simulink model "Modelo_COMPLETO_MARTIN"  (R2021a)
settings: Solver=ode15s  StartTime=0.0  StopTime=100  FixedStep=0.001  MaxStep=0.0003  RelTol=1e-3
InitFcn:
  | errordlg(DAStudio.message('Stateflow:misc:CannotSimulateWithDemoLicense'));DAStudio.error('Stateflow:misc:InvalidStateflowLicense');
model workspace (MAT data in the model file):
  socvcb = containers.Map
  socvcb.serialization.keys = {}
  socvcb.serialization.values = {}
  socvcb.serialization.uniformity = 0
  socvcb.serialization.keyType = 'double'
  socvcb.serialization.valueType = 'any'
values from neighbouring files (symbols this model uses):
  a_l_max = 0.75    [WorkspaceData.m]
  a_t_max = 0.8    [WorkspaceData.m]
  b_ah = -(b_eqh/i_h - n_h*w_posh*J_eqh/i_h)    [WorkspaceData.m]
  b_at = -double(soluc.b_at)    [WorkspaceData.m]
  b_cx = 1e6    (= 1000000)    [WorkspaceData.m]
  b_cy = 1e7    (= 10000000)    [WorkspaceData.m]
  b_hb = 1.0E+8    (= 100000000)    [WorkspaceData.m]
  b_hd = 8    [WorkspaceData.m]
  b_hEb = 2.2E+9    (= 2200000000)    [WorkspaceData.m]
  b_hm = 18    [WorkspaceData.m]
  b_t = 90    [WorkspaceData.m]
  b_tb = 5e6    (= 5000000)    [WorkspaceData.m]
  b_td = 1.8    [WorkspaceData.m]
  b_tm = 6    [WorkspaceData.m]
  b_tw = 3.0e3    (= 3000)    [WorkspaceData.m]
  b_wu = 1500    [WorkspaceData.m]
  barco_x = 0:0.01:50    [WorkspaceData.m]
  barco_y = interp1(bx_c0,by_c0,barco_x,'previous')    [WorkspaceData.m]
  carro_y = ones(1,20)*45    [WorkspaceData.m]
  constante_frenos = 10    [WorkspaceData.m]
  f = 0.1    [WorkspaceData.m]
  F_D_n_x = ones(1,5)*50    [WorkspaceData.m]
  F_D_n_y = 43:1:47    [WorkspaceData.m]
  F_D_u_x = ones(1,5)*53    [WorkspaceData.m]
  F_D_u_y = 43:1:47    [WorkspaceData.m]
  F_I_n_x = ones(1,5)*-30    [WorkspaceData.m]
  F_I_n_y = 43:1:47    [WorkspaceData.m]
  F_I_u_x = ones(1,5)*-33    [WorkspaceData.m]
  F_I_u_y = 43:1:47    [WorkspaceData.m]
  g = 9.80665    [WorkspaceData.m]
  H_c = 2.5    [WorkspaceData.m]
  i_h = 22    [WorkspaceData.m]
  i_t = 30    [WorkspaceData.m]
  J_hdhEb = 3800    [WorkspaceData.m]
  J_hmhb = 30    [WorkspaceData.m]
  J_td = 1200    [WorkspaceData.m]
  J_tmtb = 7    [WorkspaceData.m]
  K_cy = 1.8e9    (= 1800000000)    [WorkspaceData.m]
  K_sah = -n_h*w_posh^2*J_eqh/i_h    [WorkspaceData.m]
  K_sat = double(soluc.K_sat)    [WorkspaceData.m]
  K_siah = w_posh^3*J_eqh/i_h    [WorkspaceData.m]
  K_siat = -double(soluc.K_siat)    [WorkspaceData.m]
  K_tw = 4.8e5    (= 480000)    [WorkspaceData.m]
  k_wu = 2.36E+9    (= 2360000000)    [WorkspaceData.m]
  M_cmax = 70000    [WorkspaceData.m]
  M_s = 15000    [WorkspaceData.m]
  M_t = 30000    [WorkspaceData.m]
  muelle_x = -35:0.01:0    [WorkspaceData.m]
  muelle_y = interp1(mx_c0,my_c0,muelle_x,'previous')    [WorkspaceData.m]
  pos_i_lh = 45-pos_i_yl    [WorkspaceData.m]
  pos_i_x = -13.5    [WorkspaceData.m]
  pos_i_yl = Y_c0(100*(pos_i_x+30)+1)+1    [WorkspaceData.m]
  r_hd = 0.75    [WorkspaceData.m]
  r_td = 0.5    [WorkspaceData.m]
  riel_x = -35:1:55    [WorkspaceData.m]
  riel_y = ones(1,91)*45    [WorkspaceData.m]
  T_hbMax = 5e4    (= 50000)    [WorkspaceData.m]
  T_hEbMax = 1.1e6    (= 1100000)    [WorkspaceData.m]
  T_s0 = T_s1    (= 0.02)    [WorkspaceData.m]
  T_s1 = 20e-3    (= 0.02)    [WorkspaceData.m]
  T_s2 = 5e-3    (= 0.005)    [WorkspaceData.m]
  T_tbmax = 5e3    (= 5000)    [WorkspaceData.m]
  tau_hm = 1e-3    (= 0.001)    [WorkspaceData.m]
  tau_tm = 1e-3    (= 0.001)    [WorkspaceData.m]
  xx_c0 = -30:0.01:50    [WorkspaceData.m]
  Y_t0 = 45    [WorkspaceData.m]
undefined symbols (not defined in the file or in its folder): sfprivate
libraries: simulink x9, vrlib x1
PreSaveFcn:
  | errordlg(DAStudio.message('Stateflow:misc:CannotSaveWithDemoLicense'));DAStudio.error('Stateflow:misc:InvalidStateflowLicense');
settings Model: Creator=Martin Tous

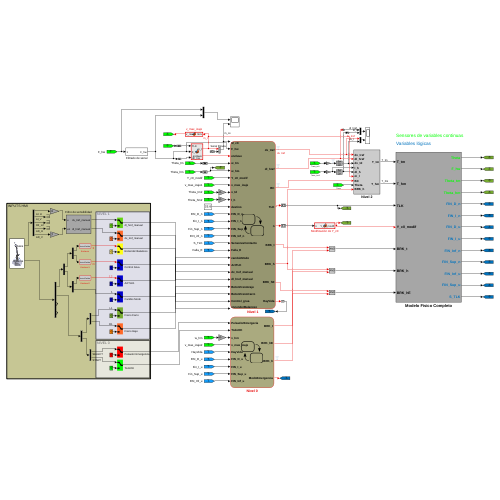
[thumbnail: Simulink's stored preview of the top-level diagram]
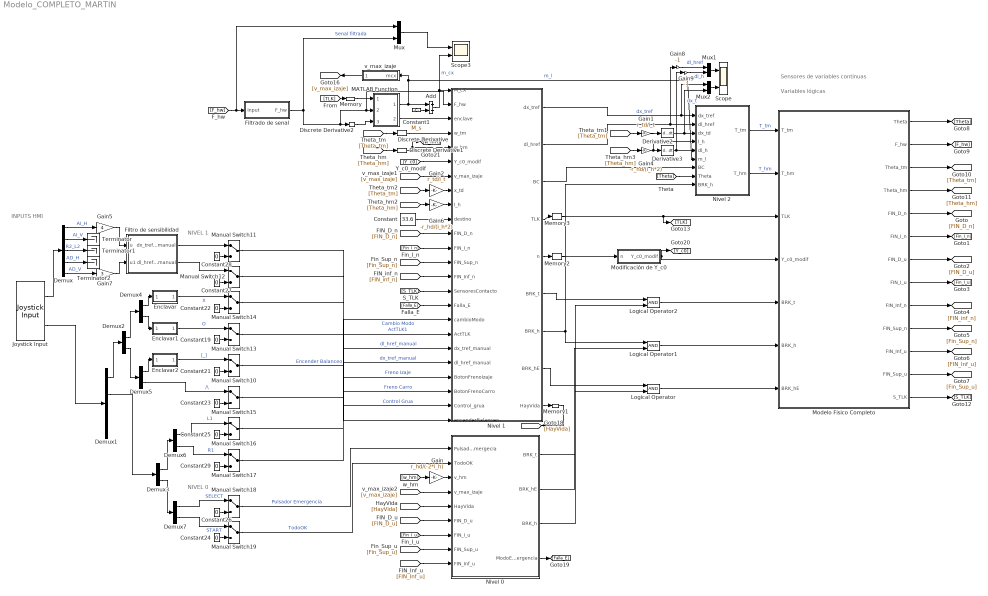
== system Modelo_COMPLETO_MARTIN ==
  note: Variables lógicas
  note: Sensores de variables continuas
  note: INPUTS HMI
  note: NIVEL 1
  note: NIVEL 0
  Add : Sum  Inputs=+-
  Constant : Constant  Value=33.6
  Constant1 : Constant  Value=M_s  SampleTime=T_s1
  Constant{19,21..23,25,27..29} (8 alike) : Constant  Value=0  SampleTime=T_s1
  Constant24 : Constant  Value=0  SampleTime=T_s0
  Constant26 : Constant  Value=0  SampleTime=T_s0
  Demux : Demux  Outputs=5
  Demux1 : Demux
  Demux{2..7} (6 alike) : Demux  Outputs=2
  Derivative2 : Derivative
  Derivative3 : Derivative
  Discrete Derivative : simulink/Discrete/Discrete Derivative  gainval=1.0  ICPrevScaledInput=0.0  OutMin=[]  OutMax=[]  OutDataType=fixdt(1, 16)  OutScaling=2^-10  DoSatur=off
  Discrete Derivative1 : simulink/Discrete/Discrete Derivative  gainval=1.0  ICPrevScaledInput=0.0  OutMin=[]  OutMax=[]  OutDataType=fixdt(1, 16)  OutScaling=2^-10  DoSatur=off
  Discrete Derivative2 : simulink/Discrete/Discrete Derivative  gainval=1.0  ICPrevScaledInput=0.0  OutMin=[]  OutMax=[]  OutDataType=fixdt(1, 16)  OutScaling=2^-10  DoSatur=off
  Enclavar : Stateflow chart  InitFcn=sfprivate('sf_demo_disclaimer');error('Preventing simulation in the absence of Stateflow license');  TreatAsAtomicUnit=on  mask(INVALID){}
      settings: PreSaveFcn=sfprivate('sf_demo_disclaimer');error('Preventing save to avoid model corruptions in the absence of Stateflow license');  OpenFcn=sfprivate('sf_demo_disclaimer');
  Enclavar1 : Stateflow chart  InitFcn=sfprivate('sf_demo_disclaimer');error('Preventing simulation in the absence of Stateflow license');  TreatAsAtomicUnit=on  mask(INVALID){}
      settings: PreSaveFcn=sfprivate('sf_demo_disclaimer');error('Preventing save to avoid model corruptions in the absence of Stateflow license');  OpenFcn=sfprivate('sf_demo_disclaimer');
  Enclavar2 : Stateflow chart  InitFcn=sfprivate('sf_demo_disclaimer');error('Preventing simulation in the absence of Stateflow license');  TreatAsAtomicUnit=on  mask(INVALID){}
      settings: PreSaveFcn=sfprivate('sf_demo_disclaimer');error('Preventing save to avoid model corruptions in the absence of Stateflow license');  OpenFcn=sfprivate('sf_demo_disclaimer');
  Filtrado de senal : Subsystem
  Filtro de sensibilidad : Subsystem
  Gain : Gain  Gain=r_hd/(-2*i_h)
  Gain1 : Gain  Gain=r_td/i_t
  Gain2 : Gain  Gain=r_td/i_t
  Gain4 : Gain  Gain=-r_hd/(i_h*2)
  Gain5 : Gain  Gain=4
  Gain6 : Gain  Gain=-r_hd/(i_h*2)
  Gain7 : Gain  Gain=3
  Gain8 : Gain  Gain=-1
  Gain9 : Gain  Gain=-1
  Joystick Input : vrlib/Joystick Input  joyid=1  adjustports=on  forcefeed=off
  Logical Operator : Logic  AllPortsSameDT=off  OutDataTypeStr=boolean
  Logical Operator1 : Logic  AllPortsSameDT=off  OutDataTypeStr=boolean
  Logical Operator2 : Logic  AllPortsSameDT=off  OutDataTypeStr=boolean
  MATLAB Function : MATLAB Function  InitFcn=sfprivate('sf_demo_disclaimer');error('Preventing simulation in the absence of Stateflow license');  TreatAsAtomicUnit=on  mask(INVALID){}
      settings: PreSaveFcn=sfprivate('sf_demo_disclaimer');error('Preventing save to avoid model corruptions in the absence of Stateflow license');  OpenFcn=sfprivate('sf_demo_disclaimer');
  Manual Switch{10..19} (10 alike) : ManualSwitch
  Memory : Memory  InheritSampleTime=on  LinearizeAsDelay=on
  Memory1 : Memory  InheritSampleTime=on
  Memory2 : Memory  InitialCondition=500  InheritSampleTime=on
  Memory3 : Memory  InheritSampleTime=on
  Modelo Fisico Completo : Subsystem
  Modificación de Y_c0 : MATLAB Function  InitFcn=sfprivate('sf_demo_disclaimer');error('Preventing simulation in the absence of Stateflow license');  TreatAsAtomicUnit=on  mask(INVALID){}
      settings: PreSaveFcn=sfprivate('sf_demo_disclaimer');error('Preventing save to avoid model corruptions in the absence of Stateflow license');  OpenFcn=sfprivate('sf_demo_disclaimer');
  Mux : Mux  Inputs=2
  Mux1 : Mux  Inputs=2
  Mux2 : Mux  Inputs=2
  Nivel 0 : Stateflow chart  InitFcn=sfprivate('sf_demo_disclaimer');error('Preventing simulation in the absence of Stateflow license');  TreatAsAtomicUnit=on  mask(INVALID){}
      settings: PreSaveFcn=sfprivate('sf_demo_disclaimer');error('Preventing save to avoid model corruptions in the absence of Stateflow license');  OpenFcn=sfprivate('sf_demo_disclaimer');  PortSchema="{\"entries\":[{\"content\":{\"sides\":[{\"content\":{\"connectorIds\":[\"In6\",\"In9\",\"In8\",\"In7\",\"In1\",\"In2\",\"In3\",\"In5\",\"In4\"]},\"type\":\"ConnectorPlacement.EquallySpacedRectSide\",\"uuid\":\"92abb5b4-7f8d-4d16-9e1c-3f1528aec02e\"},{\"content\":{\"connectorIds\":[\"Out2\",\"Out3\",\"Out1\",\"Out4\"],\"side\":\"RIGHT\"},\"type\":\"ConnectorPlacement.EquallySpacedRectSide\",\"uuid\":\"fdfc4918-925b-4492-9924-9f3ed7c6f0ea\"},{\"content\":{\"connectorIds\":[],\"side\":\"TOP\"},\"type\":\"ConnectorPlacement.EquallySpacedRectSide\",\"uuid\":\"6cd2c614-9727-439b-b51b-96ebe361e1e6\"},{\"content\":{\"connectorIds\":[],\"side\":\"BOTTOM\"},\"type\":\"ConnectorPlacement.EquallySpacedRectSide\",\"uuid\":\"c327f02f-ffd6-4494-8eea-bb6a75c04a8c\"}]},\"type\":\"ConnectorPlacement.EquallySpacedConnector\",\"uuid\":\"17c891de-27fd-4863-a62e-79c0c94ffbc9\"}],\"packageUris\":[\"http://schema.mathworks.com/mf0/Connector/R2020b\"],\"version\":\"1.0\"}"
  Nivel 1 : Stateflow chart  InitFcn=sfprivate('sf_demo_disclaimer');error('Preventing simulation in the absence of Stateflow license');  TreatAsAtomicUnit=on  mask(INVALID){}
      settings: PreSaveFcn=sfprivate('sf_demo_disclaimer');error('Preventing save to avoid model corruptions in the absence of Stateflow license');  OpenFcn=sfprivate('sf_demo_disclaimer');  PortSchema="{\"entries\":[{\"content\":{\"sides\":[{\"content\":{\"connectorIds\":[\"In1\",\"In2\",\"In23\",\"In5\",\"In4\",\"In20\",\"In13\",\"In22\",\"In21\",\"In24\",\"In7\",\"In8\",\"In10\",\"In11\",\"In3\",\"In6\",\"In19\",\"In18\",\"In9\",\"In12\",\"In15\",\"In14\",\"In16\",\"In17\"]},\"type\":\"ConnectorPlacement.EquallySpacedRectSide\",\"uuid\":\"92abb5b4-7f8d-4d16-9e1c-3f1528aec02e\"},{\"content\":{\"connectorIds\":[\"Out6\",\"Out7\",\"Out1\",\"Out8\",\"Out9\",\"Out5\",\"Out3\",\"Out4\",\"Out2\"],\"side\":\"RIGHT\"},\"type\":\"ConnectorPlacement.EquallySpacedRectSide\",\"uuid\":\"fdfc4918-925b-4492-9924-9f3ed7c6f0ea\"},{\"content\":{\"side\":\"TOP\"},\"type\":\"ConnectorPlacement.EquallySpacedRectSide\",\"uuid\":\"6cd2c614-9727-439b-b51b-96ebe361e1e6\"}]},\"type\":\"ConnectorPlacement.EquallySpacedConnector\",\"uuid\":\"17c891de-27fd-4863-a62e-79c0c94ffbc9\"}],\"packageUris\":[\"http://schema.mathworks.com/mf0/Connector/R2020b\"],\"version\":\"1.0\"}"
  Nivel 2 : Subsystem
  Scope : Scope  NumInputPorts=2
  Scope3 : Scope  NumInputPorts=2
  Terminator : Terminator
  Terminator1 : Terminator
  Terminator2 : Terminator
  v_max_izaje : MATLAB Function  InitFcn=sfprivate('sf_demo_disclaimer');error('Preventing simulation in the absence of Stateflow license');  TreatAsAtomicUnit=on  mask(INVALID){}
      settings: PreSaveFcn=sfprivate('sf_demo_disclaimer');error('Preventing save to avoid model corruptions in the absence of Stateflow license');  OpenFcn=sfprivate('sf_demo_disclaimer');
  wires:
  MATLAB Function/2(enclave) -> Nivel 1/23(enclave)
  Gain9/1 -> Mux1/2  "dl_h"
  Memory/1 -> MATLAB Function/1(TLK)
  [FIN_inf_n] -> Nivel 1/11(FIN_Inf_n)
  Mux/1 -> Scope3/1
  [Fin_Sup_n] -> Nivel 1/10(FIN_Sup_n)
  [Fin_Sup_u] -> Nivel 0/5(FIN_Sup_u)
  [FIN_Inf_u] -> Nivel 0/4(FIN_Inf_u)
  [Theta_hm] -> Gain4/1
  Modelo Fisico Completo/12(FIN_Sup_u) -> [Fin_Sup_u]
  Nivel 2/2(T_hm) -> Modelo Fisico Completo/2(T_hm)  "T_hm"
  Nivel 1/8(TLK) -> Memory3/1
  v_max_izaje/1(v_maxh) -> [v_max_izaje]
  [FIN_D_n] -> Nivel 1/7(FIN_D_n)
  [Theta_tm] -> Discrete Derivative/1
  Modelo Fisico Completo/6(FIN_I_n) -> [Fin_I_n]
  Filtrado de senal/1(F_hw) -> Nivel 1/2(F_hw), MATLAB Function/2(F_hw), Discrete Derivative2/1, Mux/2  "Senal filtrada"
  Add/1 -> Nivel 1/1(M_cX), Scope3/2  "m_cx"
  [Theta] -> Nivel 2/8(Theta)
  MATLAB Function/1(m_l) -> v_max_izaje/1(mcx), Nivel 2/6(m_l), Add/1  "m_l"
  Nivel 2/1(T_tm) -> Modelo Fisico Completo/1(T_tm)  "T_tm"
  Constant1/1 -> Add/2
  Gain6/1 -> Nivel 1/21(l_h)
  Logical Operator2/1 -> Modelo Fisico Completo/5(BRK_t)
  Discrete Derivative1/1 -> [w_hm], Nivel 1/4(w_hm)
  Nivel 1/3(BRK_h) -> Nivel 2/9(BRK_h), Logical Operator1/1
  [FIN_D_u] -> Nivel 0/2(FIN_D_u)
  Gain8/1 -> Mux1/1  "dl_href"
  Memory1/1 -> [HayVida]
  Modelo Fisico Completo/1(Theta) -> [Theta]
  [Fin_I_u] -> Nivel 0/3(FIN_I_u)
  Nivel 1/2(HayVida) -> Memory1/1
  Modelo Fisico Completo/9(FIN_Inf_n) -> [FIN_inf_n]
  Mux1/1 -> Scope/1
  Nivel 1/4(BRK_hE) -> Logical Operator/1
  Nivel 1/9(n) -> Memory2/1
  Memory2/1 -> Modificación de Y_c0/1(n)
  Gain/1 -> Nivel 0/8(v_hm)
  Nivel 0/4(ModoEmergencia) -> [Falla_E]
  Modelo Fisico Completo/8(FIN_I_u) -> [Fin_I_u]
  [Falla_E] -> Nivel 1/6(Falla_E)
  Modelo Fisico Completo/5(FIN_D_n) -> [FIN_D_n]
  [Theta_hm] -> Gain6/1
  Modelo Fisico Completo/7(FIN_D_u) -> [FIN_D_u]
  [w_hm] -> Gain/1
  [F_hw] -> Mux/1, Filtrado de senal/1(Input)
  [Fin_I_n] -> Nivel 1/8(FIN_I_n)
  Mux2/1 -> Scope/2
  [HayVida] -> Nivel 0/1(HayVida)
  Discrete Derivative2/1 -> MATLAB Function/3(dF_hw)
  [Theta_hm] -> Discrete Derivative1/1
  Modelo Fisico Completo/10(FIN_Sup_n) -> [Fin_Sup_n]
  Nivel 1/7(dl_href) -> Gain8/1, Nivel 2/2(dl_href)
  Logical Operator1/1 -> Modelo Fisico Completo/6(BRK_h)
  Nivel 0/2(BRK_t) -> Logical Operator2/2
  Memory3/1 -> [TLK], Modelo Fisico Completo/3(TLK)
  Nivel 0/1(BRK_h) -> Logical Operator/2
  [Theta_tm] -> Gain2/1
  Modelo Fisico Completo/2(F_hw) -> [F_hw]
  [Y_c0] -> Nivel 1/20(Y_c0_modif)
  Logical Operator/1 -> Modelo Fisico Completo/7(BRK_hE)
  [TLK] -> Memory/1
  Modelo Fisico Completo/4(Theta_hm) -> [Theta_hm]
  Gain1/1 -> Derivative2/1
  Nivel 1/5(BRK_t) -> Logical Operator2/1
  [S_TLK] -> Nivel 1/3(SensoresContacto)
  Modelo Fisico Completo/13(S_TLK) -> [S_TLK]
  Modelo Fisico Completo/3(Theta_tm) -> [Theta_tm]
  Modificación de Y_c0/1(Y_c0_modif) -> Modelo Fisico Completo/4(Y_c0_modif), [Y_c0]
  Discrete Derivative/1 -> Nivel 1/5(w_tm)
  Gain4/1 -> Nivel 2/4(l_h), Derivative3/1
  [v_max_izaje] -> Nivel 0/7(v_max_izaje)
  Nivel 0/3(BRK_hE) -> Logical Operator1/2
  Modelo Fisico Completo/11(FIN_Inf_u) -> [FIN_Inf_u]
  Gain2/1 -> Nivel 1/22(x_td)
  [v_max_izaje] -> Nivel 1/13(v_max_izaje)
  Nivel 1/1(BC) -> Nivel 2/7(BC)
  [Theta_tm] -> Gain1/1
  Derivative3/1 -> Gain9/1, Nivel 2/5(dl_h)
  Derivative2/1 -> Mux2/2, Nivel 2/3(dx_td)  "dx_t"
  Nivel 1/6(dx_tref) -> Mux2/1, Nivel 2/1(dx_tref)  "dx_tref"
  Manual Switch17/1 -> Nivel 1/15(BotonFrenoIzaje)  "Freno Izaje"
  Demux1/1 -> Demux2/1
  Demux2/1 -> Demux4/1
  Demux5/1 -> Enclavar2/1(boton)
  Demux/2 -> Terminator/1  "AI_V"
  Gain5/1 -> Filtro de sensibilidad/1(u)
  Demux1/2 -> Demux3/1
  Demux3/2 -> Demux7/1
  Enclavar2/1(salida) -> Manual Switch10/1  "[_]"
  Joystick Input/1 -> Demux/1
  Filtro de sensibilidad/1(dx_tref_manual) -> Manual Switch11/1
  Demux/1 -> Gain5/1  "AI_H"
  Demux4/1 -> Enclavar/1(boton)
  Manual Switch19/1 -> Nivel 0/9(TodoOK)  "TodoOK"
  Manual Switch18/1 -> Nivel 0/6(PulsadorEmergecia)  "Pulsador Emergencia"
  Constant26/1 -> Manual Switch18/2
  Demux/5 -> Gain7/1  "AD_V"
  Manual Switch14/1 -> Nivel 1/17(encenderBalanceo)  "Encender Balanceo"
  Filtro de sensibilidad/2(dl_href_manual) -> Manual Switch12/1
  Demux5/2 -> Manual Switch15/1  "/\\"
  Demux/4 -> Terminator2/1  "AD_H"
  Constant28/1 -> Manual Switch11/2
  Constant24/1 -> Manual Switch19/2
  Enclavar/1(salida) -> Manual Switch14/1  "X"
  Enclavar1/1(salida) -> Manual Switch13/1  "O"
  Demux7/2 -> Manual Switch19/1  "START"
  Demux2/2 -> Demux5/1
  Constant25/1 -> Manual Switch16/2
  Constant22/1 -> Manual Switch14/2
  Demux7/1 -> Manual Switch18/1  "SELECT"
  Constant23/1 -> Manual Switch15/2
  Constant29/1 -> Manual Switch17/2
  Demux6/2 -> Manual Switch17/1  "R1"
  Demux3/1 -> Demux6/1
  Constant27/1 -> Manual Switch12/2
  Manual Switch15/1 -> Nivel 1/19(cambioModo)  "Cambio Modo"
  Demux/3 -> Terminator1/1  "R2_L2"
  Demux6/1 -> Manual Switch16/1  "L1"
  Joystick Input/2 -> Demux1/1
  Constant19/1 -> Manual Switch13/2
  Manual Switch10/1 -> Nivel 1/18(ActTLK)  "ActTLK1"
  Manual Switch16/1 -> Nivel 1/14(BotonFrenoCarro)  "Freno Carro"
  Gain7/1 -> Filtro de sensibilidad/2(u1)
  Constant21/1 -> Manual Switch10/2
  Demux4/2 -> Enclavar1/1(boton)
  Manual Switch11/1 -> Nivel 1/9(dx_tref_manual)  "dl_href_manual"
  Manual Switch12/1 -> Nivel 1/12(dl_href_manual)  "dx_tref_manual"
  Manual Switch13/1 -> Nivel 1/16(Control_grua)  "Control Grua"
  Constant/1 -> Nivel 1/24(destino)

== system Modelo_COMPLETO_MARTIN/Filtrado de senal ==
  Input : Inport
  Leaky Integrator : Subsystem
  Moving average : Subsystem
  F_hw : Outport
  wires:
  Leaky Integrator/1(Salida) -> Moving average/1(Salida)  "pasa bajo"
  Input/1 -> Leaky Integrator/1(Entrada)  "sin filtrar"
  Moving average/1(F_hw) -> F_hw/1  "filtrada"

== system Modelo_COMPLETO_MARTIN/Filtro de sensibilidad ==
  u : Inport
  u1 : Inport  Port=2
  Compare To Constant : simulink/Logic and Bit Operations/Compare To Constant  relop=>=  const=f  OutDataTypeStr=boolean
  Compare To Constant1 : simulink/Logic and Bit Operations/Compare To Constant  relop=<=  const=-f  OutDataTypeStr=boolean
  Compare To Constant2 : simulink/Logic and Bit Operations/Compare To Constant  relop=>=  const=f  OutDataTypeStr=boolean
  Compare To Constant3 : simulink/Logic and Bit Operations/Compare To Constant  relop=<=  const=-f  OutDataTypeStr=boolean
  OR : Logic  Operator=OR  IconShape=distinctive  AllPortsSameDT=off  OutDataTypeStr=boolean
  OR1 : Logic  Operator=OR  IconShape=distinctive  AllPortsSameDT=off  OutDataTypeStr=boolean
  Product : Product
  Product1 : Product
  dx_tref_manual : Outport
  dl_href_manual : Outport  Port=2
  wires:
  u/1 -> Compare To Constant/1, Compare To Constant1/1, Product/2
  u1/1 -> Compare To Constant2/1, Compare To Constant3/1, Product1/2
  Compare To Constant1/1 -> OR/2
  Compare To Constant2/1 -> OR1/1
  Compare To Constant3/1 -> OR1/2
  OR1/1 -> Product1/1
  Compare To Constant/1 -> OR/1
  OR/1 -> Product/1
  Product/1 -> dx_tref_manual/1  "dx_tref_manual"
  Product1/1 -> dl_href_manual/1  "dl_href_manual"

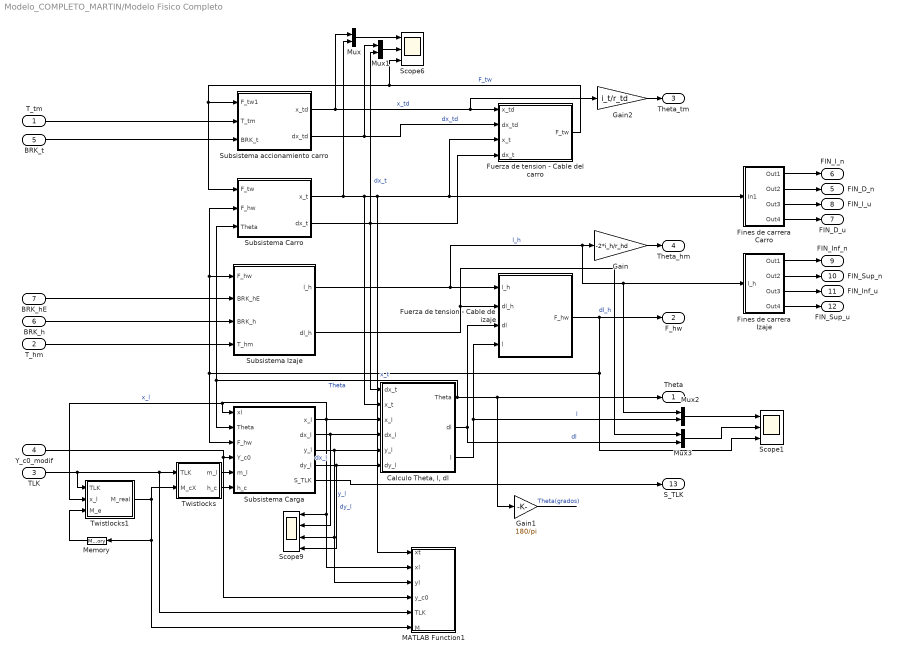
== system Modelo_COMPLETO_MARTIN/Modelo Fisico Completo ==
  T_tm : Inport
  T_hm : Inport  Port=2
  TLK : Inport  Port=3
  Y_c0_modif : Inport  Port=4
  BRK_t : Inport  Port=5
  BRK_h : Inport  Port=6
  BRK_hE : Inport  Port=7
  "Calculo Theta, l, dl" : Subsystem
  Fines de carrera Carro : Subsystem
  Fines de carrera Izaje : Subsystem
  Fuerza de tension - Cable de izaje : Subsystem
  Fuerza de tension - Cable del carro : Subsystem
  Gain : Gain  Gain=-2*i_h/r_hd
  Gain1 : Gain  Gain=180/pi
  Gain2 : Gain  Gain=i_t/r_td
  MATLAB Function1 : MATLAB Function  InitFcn=sfprivate('sf_demo_disclaimer');error('Preventing simulation in the absence of Stateflow license');  TreatAsAtomicUnit=on  mask(INVALID){}
      settings: PreSaveFcn=sfprivate('sf_demo_disclaimer');error('Preventing save to avoid model corruptions in the absence of Stateflow license');  OpenFcn=sfprivate('sf_demo_disclaimer');
  Memory : Memory  InheritSampleTime=on  LinearizeAsDelay=on
  Mux{,1..3} (4 alike) : Mux  Inputs=2
  Scope1 : Scope  NumInputPorts=3
  Scope6 : Scope  NumInputPorts=3
  Scope9 : Scope  NumInputPorts=4
  Subsistema Carga : Subsystem
  Subsistema Carro : Subsystem
  Subsistema Izaje : Subsystem
  Subsistema accionamiento carro : Subsystem
  Twistlocks : Stateflow chart  InitFcn=sfprivate('sf_demo_disclaimer');error('Preventing simulation in the absence of Stateflow license');  TreatAsAtomicUnit=on  mask(INVALID){}
      settings: PreSaveFcn=sfprivate('sf_demo_disclaimer');error('Preventing save to avoid model corruptions in the absence of Stateflow license');  OpenFcn=sfprivate('sf_demo_disclaimer');
  Twistlocks1 : Stateflow chart  InitFcn=sfprivate('sf_demo_disclaimer');error('Preventing simulation in the absence of Stateflow license');  TreatAsAtomicUnit=on  mask(INVALID){}
      settings: PreSaveFcn=sfprivate('sf_demo_disclaimer');error('Preventing save to avoid model corruptions in the absence of Stateflow license');  OpenFcn=sfprivate('sf_demo_disclaimer');  PortSchema="{\"entries\":[{\"content\":{\"sides\":[{\"content\":{\"connectorIds\":[\"In3\",\"In1\",\"In2\"]},\"type\":\"ConnectorPlacement.EquallySpacedRectSide\",\"uuid\":\"4fec8e6a-f8fa-4feb-a633-b12cd10cfa10\"},{\"content\":{\"connectorIds\":[\"Out1\"],\"side\":\"RIGHT\"},\"type\":\"ConnectorPlacement.EquallySpacedRectSide\",\"uuid\":\"3a43ccb0-d7f9-40a2-9c07-07991ad7e582\"},{\"content\":{\"connectorIds\":[],\"side\":\"TOP\"},\"type\":\"ConnectorPlacement.EquallySpacedRectSide\",\"uuid\":\"c629bb8f-87a5-4586-8b89-8bb15a2e67dc\"}]},\"type\":\"ConnectorPlacement.EquallySpacedConnector\",\"uuid\":\"e5885a79-67b0-4776-b045-dd8fc0c81e57\"}],\"packageUris\":[\"http://schema.mathworks.com/mf0/Connector/R2020b\"],\"version\":\"1.0\"}"
  Theta : Outport
  F_hw : Outport  Port=2
  Theta_tm : Outport  Port=3
  Theta_hm : Outport  Port=4
  FIN_D_n : Outport  Port=5
  FIN_I_n : Outport  Port=6
  FIN_D_u : Outport  Port=7
  FIN_I_u : Outport  Port=8
  FIN_Inf_n : Outport  Port=9
  FIN_Sup_n : Outport  Port=10
  FIN_Inf_u : Outport  Port=11
  FIN_Sup_u : Outport  Port=12
  S_TLK : Outport  Port=13
  wires:
  Fuerza de tension - Cable de izaje/1(F_hw) -> Subsistema Izaje/1(F_hw), Subsistema Carro/2(F_hw), Subsistema Carga/3(F_hw), Scope1/3, F_hw/1
  "Calculo Theta, l, dl"/1(Theta) -> Subsistema Carro/3(Theta), Subsistema Carga/2(Theta), Gain1/1, Theta/1  "Theta"
  Subsistema Izaje/2(dl_h) -> Fuerza de tension - Cable de izaje/2(dl_h), Mux3/1  "dl_h"
  Twistlocks/1(m_l) -> Subsistema Carga/5(m_l)
  "Calculo Theta, l, dl"/2(dl) -> Mux3/2, Fuerza de tension - Cable de izaje/3(dl)  "dl"
  TLK/1 -> Twistlocks/1(TLK), MATLAB Function1/5(TLK), Twistlocks1/3(TLK)
  BRK_hE/1 -> Subsistema Izaje/2(BRK_hE)
  T_hm/1 -> Subsistema Izaje/4(T_hm)
  BRK_t/1 -> Subsistema accionamiento carro/3(BRK_t)
  BRK_h/1 -> Subsistema Izaje/3(BRK_h)
  Twistlocks/2(h_c) -> Subsistema Carga/6(h_c)
  T_tm/1 -> Subsistema accionamiento carro/2(T_tm)
  Gain2/1 -> Theta_tm/1
  Subsistema Izaje/1(l_h) -> Fuerza de tension - Cable de izaje/1(l_h), Mux2/1, Fines de carrera Izaje/1(l_h), Gain/1  "l_h"
  Gain/1 -> Theta_hm/1
  "Calculo Theta, l, dl"/3(l) -> Mux2/2, Fuerza de tension - Cable de izaje/4(l)  "l"
  Twistlocks1/1(M_real) -> Memory/1, MATLAB Function1/6(M), Twistlocks/2(M_cX)
  Subsistema Carro/2(dx_t) -> Mux1/2, Fuerza de tension - Cable del carro/4(dx_t), "Calculo Theta, l, dl"/1(dx_t)  "dx_t"
  Subsistema Carga/5(S_TLK) -> S_TLK/1
  Y_c0_modif/1 -> MATLAB Function1/4(y_c0), Subsistema Carga/4(Y_c0)
  Subsistema Carro/1(x_t) -> MATLAB Function1/1(xt), Fines de carrera Carro/1(In1), Fuerza de tension - Cable del carro/3(x_t), "Calculo Theta, l, dl"/2(x_t), Mux/2  "x_t"
  Fines de carrera Carro/1(Out1) -> FIN_I_n/1
  Fines de carrera Carro/2(Out2) -> FIN_D_n/1
  Fines de carrera Carro/3(Out3) -> FIN_I_u/1
  Fines de carrera Carro/4(Out4) -> FIN_D_u/1
  Fines de carrera Izaje/1(Out1) -> FIN_Inf_n/1
  Fines de carrera Izaje/2(Out2) -> FIN_Sup_n/1
  Fines de carrera Izaje/3(Out3) -> FIN_Inf_u/1
  Fines de carrera Izaje/4(Out4) -> FIN_Sup_u/1
  Fuerza de tension - Cable del carro/1(F_tw) -> Subsistema Carro/1(F_tw), Subsistema accionamiento carro/1(F_tw1), Scope6/3  "F_tw"
  Subsistema accionamiento carro/2(dx_td) -> Mux1/1, Fuerza de tension - Cable del carro/2(dx_td)  "dx_td"
  Subsistema accionamiento carro/1(x_td) -> Gain2/1, Fuerza de tension - Cable del carro/1(x_td), Mux/1  "x_td"
  Subsistema Carga/3(y_l) -> "Calculo Theta, l, dl"/5(y_l), Scope9/3, MATLAB Function1/3(yl)  "y_l"
  Subsistema Carga/2(dx_l) -> "Calculo Theta, l, dl"/4(dx_l), Scope9/2  "dx_l"
  Subsistema Carga/4(dy_l) -> "Calculo Theta, l, dl"/6(dy_l), Scope9/4  "dy_l"
  Subsistema Carga/1(x_l) -> "Calculo Theta, l, dl"/3(x_l), Scope9/1, MATLAB Function1/2(xl), Twistlocks1/1(x_l), Subsistema Carga/1(xl)  "x_l"
  Mux/1 -> Scope6/1
  Mux1/1 -> Scope6/2
  Mux2/1 -> Scope1/1
  Mux3/1 -> Scope1/2
  Memory/1 -> Twistlocks1/2(M_e)
  Gain1/1 -> ?  "Theta(grados)"

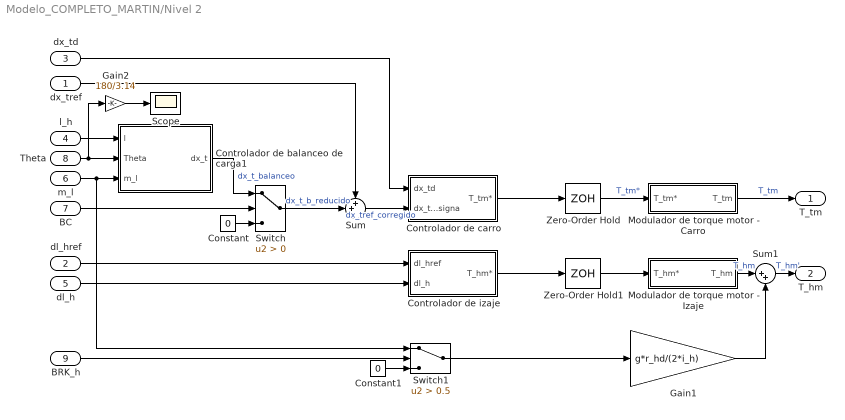
== system Modelo_COMPLETO_MARTIN/Nivel 2 ==
  dx_tref : Inport
  dl_href : Inport  Port=2
  dx_td : Inport  Port=3  SampleTime=T_s2
  l_h : Inport  Port=4  SampleTime=T_s2
  dl_h : Inport  Port=5  SampleTime=T_s2
  m_l : Inport  Port=6
  BC : Inport  Port=7
  Theta : Inport  Port=8  SampleTime=T_s2
  BRK_h : Inport  Port=9  SampleTime=T_s2
  Constant : Constant  Value=0  SampleTime=T_s2
  Constant1 : Constant  Value=0  SampleTime=T_s2
  Controlador de balanceo de carga1 : Subsystem
  Controlador de carro : Subsystem
  Controlador de izaje : Subsystem
  Gain1 : Gain  Gain=g*r_hd/(2*i_h)
  Gain2 : Gain  Gain=180/3.14
  Modulador de torque motor - Carro : Subsystem
  Modulador de torque motor - Izaje : Subsystem
  Scope : Scope
  Sum : Sum  Inputs=++|
  Sum1 : Sum  Inputs=|++
  Switch : Switch  Criteria=u2 > Threshold
  Switch1 : Switch  Criteria=u2 > Threshold  Threshold=0.5
  Zero-Order Hold : ZeroOrderHold  SampleTime=T_s2
  Zero-Order Hold1 : ZeroOrderHold  SampleTime=T_s2
  T_tm : Outport
  T_hm : Outport  Port=2
  wires:
  Sum1/1 -> T_hm/1  "T_hm'"
  Zero-Order Hold/1 -> Modulador de torque motor - Carro/1(T_tm*)  "T_tm*"
  Zero-Order Hold1/1 -> Modulador de torque motor - Izaje/1(T_hm*)
  Modulador de torque motor - Carro/1(T_tm) -> T_tm/1  "T_tm"
  Modulador de torque motor - Izaje/1(T_hm) -> Sum1/1  "T_hm"
  dx_td/1 -> Controlador de carro/1(dx_td)
  Gain2/1 -> Scope/1
  Controlador de balanceo de carga1/1(dx_t) -> Switch/1  "dx_t_balanceo"
  Theta/1 -> Controlador de balanceo de carga1/2(Theta), Gain2/1
  dx_tref/1 -> Sum/1
  Constant/1 -> Switch/3
  dl_h/1 -> Controlador de izaje/2(dl_h)
  Sum/1 -> Controlador de carro/2(dx_t_consigna)  "dx_tref_corregido"
  BC/1 -> Switch/2
  l_h/1 -> Controlador de balanceo de carga1/1(l)
  Switch/1 -> Sum/2  "dx_t_b_reducido"
  Controlador de carro/1(T_tm*) -> Zero-Order Hold/1
  Controlador de izaje/1(T_hm*) -> Zero-Order Hold1/1
  Switch1/1 -> Gain1/1
  m_l/1 -> Controlador de balanceo de carga1/3(m_l), Switch1/1
  dl_href/1 -> Controlador de izaje/1(dl_href)
  Gain1/1 -> Sum1/2
  Constant1/1 -> Switch1/3
  BRK_h/1 -> Switch1/2

== system Modelo_COMPLETO_MARTIN/Filtrado de senal/Leaky Integrator ==
  Entrada : Inport
  Constant17 : Constant
  Constant21 : Constant
  Delay1 : Delay  DelayLength=1  InitialCondition=0
  Divide1 : Product  Inputs=*/
  M : Constant  Value=100
  Product2 : Product
  Product3 : Product
  Sum3 : Sum  Inputs=-+
  Sum4 : Sum  Inputs=+-
  Sum5 : Sum  Inputs=|++
  Salida : Outport
  wires:
  Sum5/1 -> Salida/1, Delay1/1
  M/1 -> Divide1/2, Sum3/2
  Constant21/1 -> Sum4/1
  Sum4/1 -> Product2/2
  Product2/1 -> Sum5/1
  Delay1/1 -> Product3/1
  Constant17/1 -> Sum3/1
  Divide1/1 -> Product3/2, Sum4/2  "lambda"
  Product3/1 -> Sum5/2
  Sum3/1 -> Divide1/1
  Entrada/1 -> Product2/1

== system Modelo_COMPLETO_MARTIN/Filtrado de senal/Moving average ==
  Salida : Inport
  Divide : Product  Inputs=*/
  Sum of Elements : Sum  Inputs=+
  Tapped Delay : simulink/Discrete/Tapped Delay  vinit=0.0  samptime=T_s1  NumDelays=90  DelayOrder=Oldest  includeCurrent=off
  Vector Concatenate : Concatenate
  Width : Width
  F_hw : Outport
  wires:
  Width/1 -> Divide/2
  Tapped Delay/1 -> Vector Concatenate/2
  Vector Concatenate/1 -> Width/1, Sum of Elements/1
  Salida/1 -> Tapped Delay/1, Vector Concatenate/1
  Divide/1 -> F_hw/1
  Sum of Elements/1 -> Divide/1

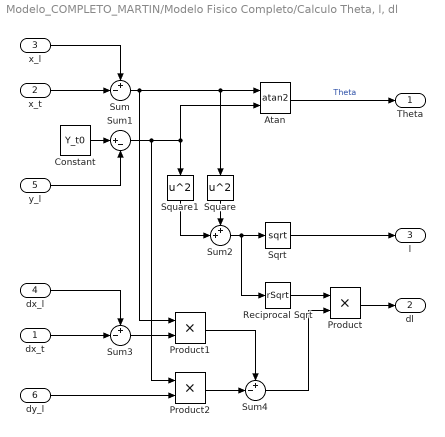
== system Modelo_COMPLETO_MARTIN/Modelo Fisico Completo/Calculo Theta, l, dl ==
  dx_t : Inport
  x_t : Inport  Port=2
  x_l : Inport  Port=3
  dx_l : Inport  Port=4
  y_l : Inport  Port=5
  dy_l : Inport  Port=6
  Atan : Trigonometry  Operator=atan2
  Constant : Constant  Value=Y_t0
  Product : Product
  Product1 : Product
  Product2 : Product
  Reciprocal Sqrt : Sqrt  Operator=rSqrt  SaturateOnIntegerOverflow=on
  Sqrt : Sqrt  SaturateOnIntegerOverflow=on
  Square : Math  Operator=square  SaturateOnIntegerOverflow=on
  Square1 : Math  Operator=square  SaturateOnIntegerOverflow=on
  Sum : Sum  Inputs=+-|
  Sum1 : Sum  Inputs=|+-
  Sum2 : Sum  Inputs=++|
  Sum3 : Sum  Inputs=+-|
  Sum4 : Sum  Inputs=+-|
  Theta : Outport
  dl : Outport  Port=2
  l : Outport  Port=3
  wires:
  y_l/1 -> Sum1/2
  Sum1/1 -> Product2/1, Square1/1, Atan/2
  Sum/1 -> Square/1, Atan/1, Product1/1
  Constant/1 -> Sum1/1
  Atan/1 -> Theta/1  "Theta"
  x_l/1 -> Sum/1
  x_t/1 -> Sum/2
  Square/1 -> Sum2/1
  Square1/1 -> Sum2/2
  Sum2/1 -> Reciprocal Sqrt/1, Sqrt/1
  Sqrt/1 -> l/1
  Reciprocal Sqrt/1 -> Product/1
  dx_l/1 -> Sum3/1
  dx_t/1 -> Sum3/2
  Sum3/1 -> Product1/2
  Product1/1 -> Sum4/1
  dy_l/1 -> Product2/2
  Product2/1 -> Sum4/2
  Sum4/1 -> Product/2
  Product/1 -> dl/1

== system Modelo_COMPLETO_MARTIN/Modelo Fisico Completo/Fines de carrera Carro ==
  In1 : Inport
  Constant1 : Constant  Value=53
  Constant2 : Constant  Value=50
  Constant3 : Constant  Value=-30
  Constant7 : Constant  Value=-33
  GreaterThan1 : RelationalOperator  OutDataTypeStr=boolean  RndMeth=Simplest
  GreaterThan2 : RelationalOperator  Operator=<=  OutDataTypeStr=boolean  RndMeth=Simplest
  GreaterThan5 : RelationalOperator  OutDataTypeStr=boolean  RndMeth=Simplest
  GreaterThan6 : RelationalOperator  Operator=<=  OutDataTypeStr=boolean  RndMeth=Simplest
  Out1 : Outport
  Out2 : Outport  Port=2
  Out3 : Outport  Port=3
  Out4 : Outport  Port=4
  wires:
  GreaterThan1/1 -> Out2/1
  In1/1 -> GreaterThan5/1, GreaterThan6/1, GreaterThan1/1, GreaterThan2/1
  GreaterThan2/1 -> Out1/1
  Constant3/1 -> GreaterThan2/2
  Constant2/1 -> GreaterThan1/2
  Constant1/1 -> GreaterThan5/2
  Constant7/1 -> GreaterThan6/2
  GreaterThan6/1 -> Out3/1
  GreaterThan5/1 -> Out4/1

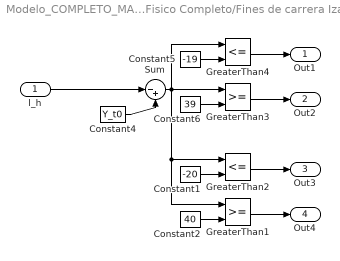
== system Modelo_COMPLETO_MARTIN/Modelo Fisico Completo/Fines de carrera Izaje ==
  l_h : Inport
  Constant1 : Constant  Value=-20
  Constant2 : Constant  Value=40
  Constant4 : Constant  Value=Y_t0
  Constant5 : Constant  Value=-19
  Constant6 : Constant  Value=39
  GreaterThan1 : RelationalOperator  OutDataTypeStr=boolean  RndMeth=Simplest
  GreaterThan2 : RelationalOperator  Operator=<=  OutDataTypeStr=boolean  RndMeth=Simplest
  GreaterThan3 : RelationalOperator  OutDataTypeStr=boolean  RndMeth=Simplest
  GreaterThan4 : RelationalOperator  Operator=<=  OutDataTypeStr=boolean  RndMeth=Simplest
  Sum : Sum  Inputs=|-+
  Out1 : Outport
  Out2 : Outport  Port=2
  Out3 : Outport  Port=3
  Out4 : Outport  Port=4
  wires:
  Constant1/1 -> GreaterThan2/2
  Sum/1 -> GreaterThan3/1, GreaterThan4/1, GreaterThan1/1, GreaterThan2/1
  Constant6/1 -> GreaterThan3/2
  Constant4/1 -> Sum/2
  Constant5/1 -> GreaterThan4/2
  Constant2/1 -> GreaterThan1/2
  GreaterThan3/1 -> Out2/1
  GreaterThan4/1 -> Out1/1
  l_h/1 -> Sum/1
  GreaterThan2/1 -> Out3/1
  GreaterThan1/1 -> Out4/1

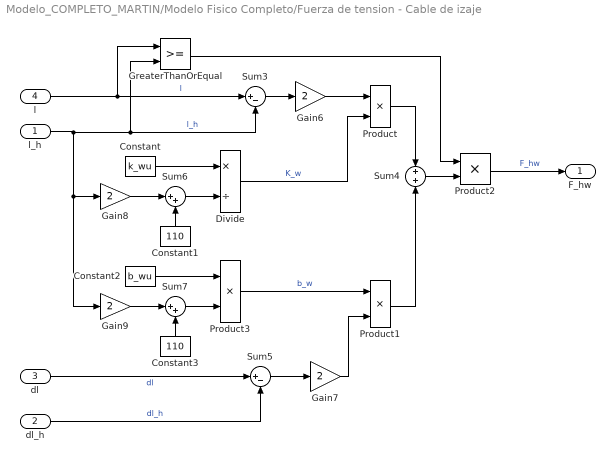
== system Modelo_COMPLETO_MARTIN/Modelo Fisico Completo/Fuerza de tension - Cable de izaje ==
  l_h : Inport
  dl_h : Inport  Port=2
  dl : Inport  Port=3
  l : Inport  Port=4
  Constant : Constant  Value=k_wu  SampleTime=[0, 0]
  Constant1 : Constant  Value=110
  Constant2 : Constant  Value=b_wu
  Constant3 : Constant  Value=110
  Divide : Product  Inputs=*/
  Gain{6..9} (4 alike) : Gain  Gain=2
  GreaterThanOrEqual : RelationalOperator  OutDataTypeStr=boolean  RndMeth=Simplest
  Product{,1..3} (4 alike) : Product
  Sum3 : Sum  Inputs=|+-
  Sum4 : Sum  Inputs=+|+
  Sum5 : Sum  Inputs=|+-
  Sum6 : Sum  Inputs=|++
  Sum7 : Sum  Inputs=|++
  F_hw : Outport
  wires:
  Sum4/1 -> Product2/2
  l_h/1 -> Sum3/2, GreaterThanOrEqual/2, Gain9/1, Gain8/1  "l_h"
  Product/1 -> Sum4/1
  Sum3/1 -> Gain6/1
  Constant1/1 -> Sum6/2
  Sum6/1 -> Divide/2
  Gain6/1 -> Product/1
  l/1 -> Sum3/1, GreaterThanOrEqual/1  "l"
  Constant/1 -> Divide/1
  dl_h/1 -> Sum5/2  "dl_h"
  Sum5/1 -> Gain7/1
  Product1/1 -> Sum4/2
  GreaterThanOrEqual/1 -> Product2/1
  Product2/1 -> F_hw/1  "F_hw"
  Constant2/1 -> Product3/1
  Divide/1 -> Product/2  "K_w"
  Gain8/1 -> Sum6/1
  Constant3/1 -> Sum7/2
  Gain9/1 -> Sum7/1
  Sum7/1 -> Product3/2
  dl/1 -> Sum5/1  "dl"
  Product3/1 -> Product1/1  "b_w"
  Gain7/1 -> Product1/2

== system Modelo_COMPLETO_MARTIN/Modelo Fisico Completo/Fuerza de tension - Cable del carro ==
  x_td : Inport
  dx_td : Inport  Port=2
  x_t : Inport  Port=3
  dx_t : Inport  Port=4
  Gain3 : Gain  Gain=K_tw
  Gain4 : Gain  Gain=b_tw
  Sum1 : Sum  Inputs=-+|
  Sum2 : Sum  Inputs=|+-
  Sum3 : Sum  Inputs=+|+
  F_tw : Outport
  wires:
  Gain4/1 -> Sum3/2
  x_t/1 -> Sum1/1
  dx_t/1 -> Sum2/2
  dx_td/1 -> Sum2/1
  Gain3/1 -> Sum3/1
  Sum1/1 -> Gain3/1
  Sum2/1 -> Gain4/1
  x_td/1 -> Sum1/2
  Sum3/1 -> F_tw/1

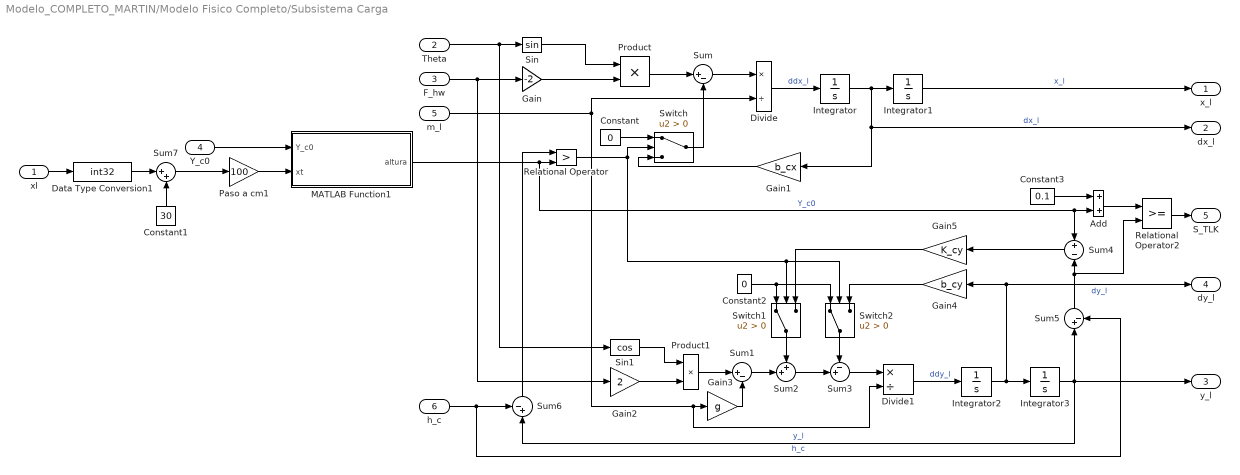
== system Modelo_COMPLETO_MARTIN/Modelo Fisico Completo/Subsistema Carga ==
  xl : Inport
  Theta : Inport  Port=2
  F_hw : Inport  Port=3
  Y_c0 : Inport  Port=4
  m_l : Inport  Port=5
  h_c : Inport  Port=6
  Add : Sum
  Constant : Constant  Value=0
  Constant1 : Constant  Value=30
  Constant2 : Constant  Value=0
  Constant3 : Constant  Value=0.1
  Data Type Conversion1 : DataTypeConversion  OutDataTypeStr=int32
  Divide : Product  Inputs=*/
  Divide1 : Product  Inputs=*/
  Gain : Gain  Gain=-2
  Gain1 : Gain  Gain=b_cx
  Gain2 : Gain  Gain=2
  Gain3 : Gain  Gain=g
  Gain4 : Gain  Gain=b_cy
  Gain5 : Gain  Gain=K_cy
  Integrator : Integrator
  Integrator1 : Integrator  InitialCondition=pos_i_x
  Integrator2 : Integrator
  Integrator3 : Integrator  InitialCondition=pos_i_yl
  MATLAB Function1 : MATLAB Function  InitFcn=sfprivate('sf_demo_disclaimer');error('Preventing simulation in the absence of Stateflow license');  TreatAsAtomicUnit=on  mask(INVALID){}
      settings: PreSaveFcn=sfprivate('sf_demo_disclaimer');error('Preventing save to avoid model corruptions in the absence of Stateflow license');  OpenFcn=sfprivate('sf_demo_disclaimer');
  Paso a cm1 : Gain  Gain=100
  Product : Product
  Product1 : Product
  Relational Operator : RelationalOperator  Operator=>  OutDataTypeStr=boolean  RndMeth=Simplest
  Relational Operator2 : RelationalOperator  OutDataTypeStr=boolean  RndMeth=Simplest
  Sin : Trigonometry
  Sin1 : Trigonometry  Operator=cos
  Sum : Sum  Inputs=|+-
  Sum1 : Sum  Inputs=|+-
  Sum2 : Sum  Inputs=++|
  Sum3 : Sum  Inputs=-+|
  Sum4 : Sum  Inputs=+|-
  Sum5 : Sum  Inputs=|+-
  Sum6 : Sum  Inputs=-+|
  Sum7 : Sum  Inputs=|++
  Switch : Switch  Criteria=u2 > Threshold
  Switch1 : Switch  Criteria=u2 > Threshold
  Switch2 : Switch  Criteria=u2 > Threshold
  x_l : Outport
  dx_l : Outport  Port=2
  y_l : Outport  Port=3
  dy_l : Outport  Port=4
  S_TLK : Outport  Port=5
  wires:
  Integrator3/1 -> y_l/1, Sum6/2, Sum5/1  "y_l"
  Relational Operator/1 -> Switch2/2, Switch1/2, Switch/2
  Divide/1 -> Integrator/1  "ddx_l"
  Switch2/1 -> Sum3/1
  Integrator/1 -> dx_l/1, Gain1/1, Integrator1/1  "dx_l"
  h_c/1 -> Sum5/2, Sum6/1  "h_c"
  Gain3/1 -> Sum1/2
  F_hw/1 -> Gain/1, Gain2/1
  Product/1 -> Sum/1
  Switch1/1 -> Sum2/1
  Sum6/1 -> Relational Operator/1
  Sum1/1 -> Sum2/2
  Gain1/1 -> Switch/3
  Integrator2/1 -> dy_l/1, Gain4/1, Integrator3/1  "dy_l"
  Gain/1 -> Product/2
  Gain5/1 -> Switch1/3
  Sin1/1 -> Product1/1
  Sin/1 -> Product/1
  Sum/1 -> Divide/1
  Integrator1/1 -> x_l/1  "x_l"
  Gain4/1 -> Switch2/3
  Sum5/1 -> Relational Operator2/2, Sum4/2
  Sum4/1 -> Gain5/1
  Theta/1 -> Sin/1, Sin1/1
  Constant2/1 -> Switch2/1, Switch1/1
  Divide1/1 -> Integrator2/1  "ddy_l"
  Gain2/1 -> Product1/2
  Product1/1 -> Sum1/1
  m_l/1 -> Divide/2, Divide1/2, Gain3/1
  Sum2/1 -> Sum3/2
  Sum3/1 -> Divide1/1
  Constant/1 -> Switch/1
  Switch/1 -> Sum/2
  MATLAB Function1/1(altura) -> Sum4/1, Add/2, Relational Operator/2  "Y_c0"
  Relational Operator2/1 -> S_TLK/1
  Paso a cm1/1 -> MATLAB Function1/2(xt)
  Y_c0/1 -> MATLAB Function1/1(Y_c0)
  xl/1 -> Data Type Conversion1/1
  Sum7/1 -> Paso a cm1/1
  Constant1/1 -> Sum7/2
  Data Type Conversion1/1 -> Sum7/1
  Add/1 -> Relational Operator2/1
  Constant3/1 -> Add/1

== system Modelo_COMPLETO_MARTIN/Modelo Fisico Completo/Subsistema Carro ==
  F_tw : Inport
  F_hw : Inport  Port=2
  Theta : Inport  Port=3
  Gain : Gain  Gain=1/M_t
  Gain1 : Gain  Gain=-b_t
  Gain2 : Gain  Gain=2
  Integrator : Integrator
  Integrator1 : Integrator  InitialCondition=pos_i_x
  Product : Product
  Sin : Trigonometry
  Sum : Sum  Inputs=+++
  x_t : Outport
  dx_t : Outport  Port=2
  wires:
  Sin/1 -> Product/1
  Gain2/1 -> Product/2
  F_hw/1 -> Gain2/1
  Integrator/1 -> Integrator1/1, dx_t/1, Gain1/1  "dx_t"
  Gain1/1 -> Sum/1
  Integrator1/1 -> x_t/1  "x_t"
  Product/1 -> Sum/2
  Gain/1 -> Integrator/1  "ddx_t"
  Sum/1 -> Gain/1
  Theta/1 -> Sin/1
  F_tw/1 -> Sum/3

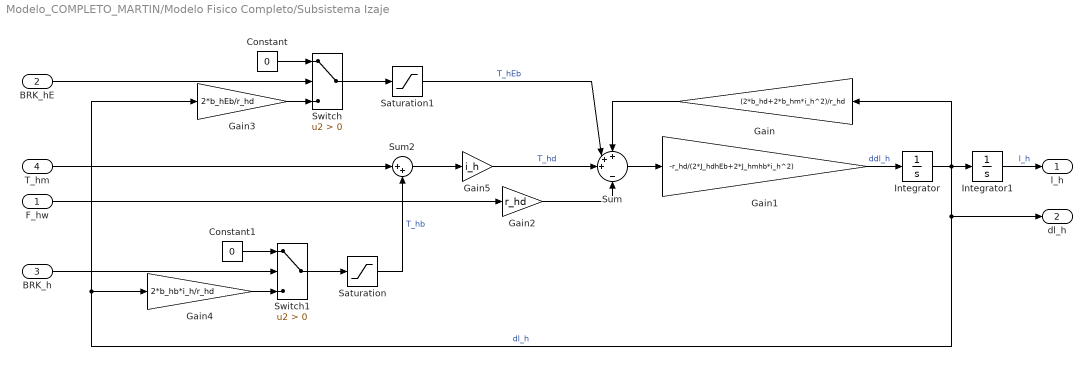
== system Modelo_COMPLETO_MARTIN/Modelo Fisico Completo/Subsistema Izaje ==
  F_hw : Inport
  BRK_hE : Inport  Port=2
  BRK_h : Inport  Port=3
  T_hm : Inport  Port=4
  Constant : Constant  Value=0
  Constant1 : Constant  Value=0
  Gain : Gain  Gain=(2*b_hd+2*b_hm*i_h^2)/r_hd
  Gain1 : Gain  Gain=-r_hd/(2*J_hdhEb+2*J_hmhb*i_h^2)
  Gain2 : Gain  Gain=r_hd
  Gain3 : Gain  Gain=2*b_hEb/r_hd
  Gain4 : Gain  Gain=2*b_hb*i_h/r_hd
  Gain5 : Gain  Gain=i_h
  Integrator : Integrator
  Integrator1 : Integrator  InitialCondition=pos_i_lh
  Saturation : Saturate  UpperLimit=T_hbMax*constante_frenos  LowerLimit=-T_hbMax*constante_frenos
  Saturation1 : Saturate  UpperLimit=T_hEbMax*constante_frenos  LowerLimit=-T_hEbMax*constante_frenos  LinearizeAsGain=off
  Sum : Sum  Inputs=+++|-
  Sum2 : Sum  Inputs=|++
  Switch : Switch  Criteria=u2 > Threshold
  Switch1 : Switch  Criteria=u2 > Threshold
  l_h : Outport
  dl_h : Outport  Port=2
  wires:
  T_hm/1 -> Sum2/1
  Saturation1/1 -> Sum/2  "T_hEb"
  Gain/1 -> Sum/1
  Gain1/1 -> Integrator/1  "ddl_h"
  Sum/1 -> Gain1/1
  Gain5/1 -> Sum/3  "T_hd"
  Integrator1/1 -> l_h/1  "l_h"
  Sum2/1 -> Gain5/1
  F_hw/1 -> Gain2/1
  Switch/1 -> Saturation1/1
  Saturation/1 -> Sum2/2  "T_hb"
  Gain2/1 -> Sum/4
  Integrator/1 -> dl_h/1, Gain3/1, Gain4/1, Gain/1, Integrator1/1  "dl_h"
  BRK_hE/1 -> Switch/2
  Gain3/1 -> Switch/3
  Constant/1 -> Switch/1
  Constant1/1 -> Switch1/1
  BRK_h/1 -> Switch1/2
  Gain4/1 -> Switch1/3
  Switch1/1 -> Saturation/1

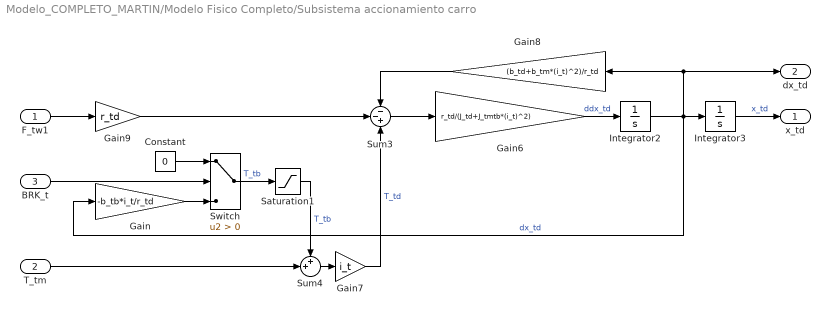
== system Modelo_COMPLETO_MARTIN/Modelo Fisico Completo/Subsistema accionamiento carro ==
  F_tw1 : Inport
  T_tm : Inport  Port=2
  BRK_t : Inport  Port=3
  Constant : Constant  Value=0
  Gain : Gain  Gain=-b_tb*i_t/r_td
  Gain6 : Gain  Gain=r_td/(J_td+J_tmtb*(i_t)^2)
  Gain7 : Gain  Gain=i_t
  Gain8 : Gain  Gain=(b_td+b_tm*(i_t)^2)/r_td
  Gain9 : Gain  Gain=r_td
  Integrator2 : Integrator
  Integrator3 : Integrator  InitialCondition=pos_i_x
  Saturation1 : Saturate  UpperLimit=T_tbmax*constante_frenos  LowerLimit=-T_tbmax*constante_frenos
  Sum3 : Sum  Inputs=--+
  Sum4 : Sum  Inputs=++|
  Switch : Switch  Criteria=u2 > Threshold
  x_td : Outport
  dx_td : Outport  Port=2
  wires:
  Switch/1 -> Saturation1/1  "T_tb"
  F_tw1/1 -> Gain9/1
  Sum3/1 -> Gain6/1
  Gain7/1 -> Sum3/3  "T_td"
  Gain8/1 -> Sum3/1
  Integrator2/1 -> Gain8/1, dx_td/1, Gain/1, Integrator3/1  "dx_td"
  Sum4/1 -> Gain7/1
  Gain6/1 -> Integrator2/1  "ddx_td"
  Gain9/1 -> Sum3/2
  T_tm/1 -> Sum4/2
  Integrator3/1 -> x_td/1  "x_td"
  Constant/1 -> Switch/1
  Gain/1 -> Switch/3
  BRK_t/1 -> Switch/2
  Saturation1/1 -> Sum4/1  "T_tb"

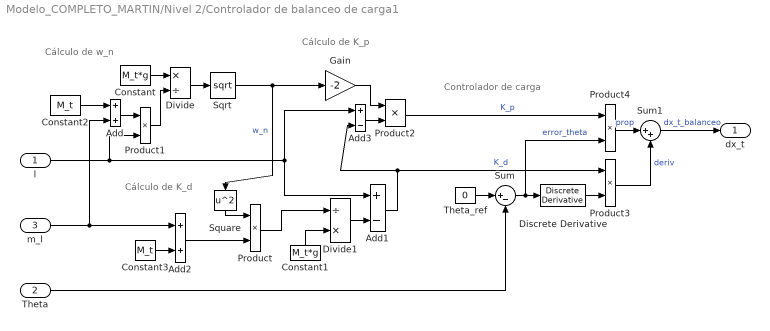
== system Modelo_COMPLETO_MARTIN/Nivel 2/Controlador de balanceo de carga1 ==
  note: Cálculo de K_p
  note: Cálculo de w_n
  note: Controlador de carga
  note: Cálculo de K_d
  l : Inport
  Theta : Inport  Port=2
  m_l : Inport  Port=3
  Add : Sum
  Add1 : Sum  Inputs=+-
  Add2 : Sum
  Add3 : Sum  Inputs=+-
  Constant : Constant  Value=M_t*g  SampleTime=T_s2
  Constant1 : Constant  Value=M_t*g  SampleTime=T_s2
  Constant2 : Constant  Value=M_t  SampleTime=T_s2
  Constant3 : Constant  Value=M_t  SampleTime=T_s2
  Discrete Derivative : simulink/Discrete/Discrete Derivative  gainval=1.0  ICPrevScaledInput=0.0  OutMin=[]  OutMax=[]  OutDataType=fixdt(1, 16)  OutScaling=2^-10  DoSatur=off
  Divide : Product  Inputs=*/
  Divide1 : Product  Inputs=/*
  Gain : Gain  Gain=-2
  Product{,1..4} (5 alike) : Product
  Sqrt : Sqrt  SaturateOnIntegerOverflow=on
  Square : Math  Operator=square  SaturateOnIntegerOverflow=on
  Sum : Sum  Inputs=|+-
  Sum1 : Sum  Inputs=|++
  Theta_ref : Constant  Value=0  SampleTime=T_s2
  dx_t : Outport
  wires:
  Theta/1 -> Sum/2
  Gain/1 -> Product2/1
  l/1 -> Add3/1, Add1/1, Product1/2
  Theta_ref/1 -> Sum/1
  Product/1 -> Divide1/1
  Constant3/1 -> Add2/2
  Sum1/1 -> dx_t/1  "dx_t_balanceo"
  Sum/1 -> Product4/2, Discrete Derivative/1  "error_theta"
  m_l/1 -> Add2/1, Add/2
  Add3/1 -> Product2/2
  Constant2/1 -> Add/1
  Add1/1 -> Product3/1, Add3/2  "K_d"
  Product4/1 -> Sum1/1  "prop"
  Add/1 -> Product1/1
  Product3/1 -> Sum1/2  "deriv"
  Square/1 -> Product/1
  Constant1/1 -> Divide1/2
  Divide1/1 -> Add1/2
  Product2/1 -> Product4/1  "K_p"
  Divide/1 -> Sqrt/1
  Constant/1 -> Divide/1
  Product1/1 -> Divide/2
  Add2/1 -> Product/2
  Discrete Derivative/1 -> Product3/2
  Sqrt/1 -> Gain/1, Square/1  "w_n"

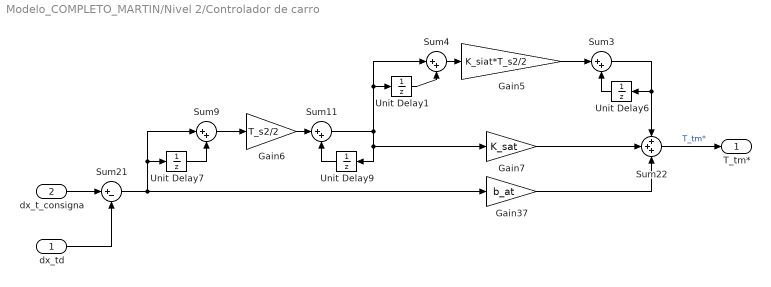
== system Modelo_COMPLETO_MARTIN/Nivel 2/Controlador de carro ==
  dx_td : Inport
  dx_t_consigna : Inport  Port=2
  Gain37 : Gain  Gain=b_at
  Gain5 : Gain  Gain=K_siat*T_s2/2
  Gain6 : Gain  Gain=T_s2/2
  Gain7 : Gain  Gain=K_sat
  Sum{3..4,9,11} (4 alike) : Sum  Inputs=|++
  Sum21 : Sum  Inputs=|+-
  Sum22 : Sum  Inputs=+++
  Unit Delay{1,6..7,9} (4 alike) : UnitDelay  SampleTime=-1  HasFrameUpgradeWarning=on
  T_tm* : Outport
  wires:
  Gain6/1 -> Sum11/1
  Sum4/1 -> Gain5/1
  Sum3/1 -> Sum22/1, Unit Delay6/1
  Unit Delay9/1 -> Sum11/2
  Gain7/1 -> Sum22/2
  Unit Delay7/1 -> Sum9/2
  Sum21/1 -> Unit Delay7/1, Sum9/1, Gain37/1
  dx_t_consigna/1 -> Sum21/1
  Sum9/1 -> Gain6/1
  Unit Delay6/1 -> Sum3/2
  Sum11/1 -> Gain7/1, Unit Delay9/1, Unit Delay1/1, Sum4/1
  Unit Delay1/1 -> Sum4/2
  Gain37/1 -> Sum22/3
  Sum22/1 -> T_tm*/1  "T_tm*"
  Gain5/1 -> Sum3/1
  dx_td/1 -> Sum21/2

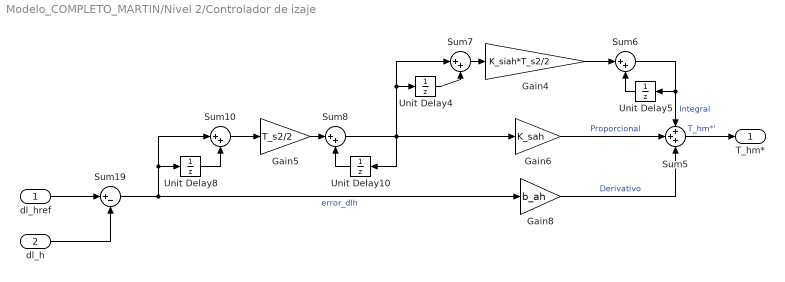
== system Modelo_COMPLETO_MARTIN/Nivel 2/Controlador de izaje ==
  dl_href : Inport
  dl_h : Inport  Port=2
  Gain4 : Gain  Gain=K_siah*T_s2/2
  Gain5 : Gain  Gain=T_s2/2
  Gain6 : Gain  Gain=K_sah
  Gain8 : Gain  Gain=b_ah
  Sum{6..8,10} (4 alike) : Sum  Inputs=|++
  Sum19 : Sum  Inputs=|+-
  Sum5 : Sum  Inputs=+++
  Unit Delay{4..5,8,10} (4 alike) : UnitDelay  SampleTime=-1  HasFrameUpgradeWarning=on
  T_hm* : Outport
  wires:
  Sum10/1 -> Gain5/1
  Gain8/1 -> Sum5/3  "Derivativo"
  Unit Delay8/1 -> Sum10/2
  Gain6/1 -> Sum5/2  "Proporcional"
  Sum8/1 -> Gain6/1, Unit Delay10/1, Unit Delay4/1, Sum7/1
  Gain5/1 -> Sum8/1
  Gain4/1 -> Sum6/1
  Unit Delay5/1 -> Sum6/2
  Sum7/1 -> Gain4/1
  Unit Delay4/1 -> Sum7/2
  Sum19/1 -> Gain8/1, Sum10/1, Unit Delay8/1  "error_dlh"
  Unit Delay10/1 -> Sum8/2
  Sum6/1 -> Sum5/1, Unit Delay5/1  "Integral"
  dl_href/1 -> Sum19/1
  dl_h/1 -> Sum19/2
  Sum5/1 -> T_hm*/1  "T_hm*'"

== system Modelo_COMPLETO_MARTIN/Nivel 2/Modulador de torque motor - Carro ==
  T_tm* : Inport
  Transfer Fcn : TransferFcn  Denominator=[tau_tm 1]
  T_tm : Outport
  wires:
  Transfer Fcn/1 -> T_tm/1
  T_tm*/1 -> Transfer Fcn/1

== system Modelo_COMPLETO_MARTIN/Nivel 2/Modulador de torque motor - Izaje ==
  T_hm* : Inport
  Transfer Fcn1 : TransferFcn  Denominator=[tau_hm 1]
  T_hm : Outport
  wires:
  T_hm*/1 -> Transfer Fcn1/1
  Transfer Fcn1/1 -> T_hm/1
